simulink model "simrotor1"  (Simulink 10.0)
settings: Solver=ode23tb  StartTime=0.0  StopTime=10.0  RelTol=1e-1  AbsTol=1e-1
undefined symbols (not defined in the file): ar, br, cr, dr, full
libraries: simulink3 x1
settings Model: Creator=bhisma  LastModifiedBy=bhisma  ExtModeTrigMode=oneshot  ExtModeArmWhenConnect=off
settings DataIOCC: SignalLoggingSaveFormat=ModelDataLogs
settings OptimizationCC: BlockReduction=off  BooleanDataType=off  LifeSpan=auto
settings DebuggingCC: SaveWithParameterizedLinksMsg=none  SignalResolutionControl=TryResolveAllWithWarning  MultiTaskDSMMsg=warning  MultiTaskCondExecSysMsg=none  SFUnexpectedBacktrackingDiag=error  SFNoUnconditionalDefaultTransitionDiag=error  SFExecutionAtInitializationDiag=warning  ArithmeticOperatorsInVariantConditions=error
settings HardwareCC: ProdBitPerPointer=64  ProdBitPerSizeT=64  ProdBitPerPtrDiffT=64  ProdLargestAtomicFloat=Float  ProdIntDivRoundTo=Zero  ProdEndianess=LittleEndian  ProdWordSize=64  ProdHWDeviceType=Intel->x86-64 (Windows64)  TargetUnknown=on
settings SFSimCC: SimUseLocalCustomCode=on  CustomCodeUndefinedFunction=FilterOut
settings RTWCC: RTWUseLocalCustomCode=on
settings CodeAppCC: StateflowObjectComments=off
settings GRTTargetCC: TargetLangStandard=C99 (ISO)
settings ConfigComp: CovMetricSettings=dwe  CovHtmlReporting=off  CovSaveCumulativeToWorkspaceVar=off  CovSaveSingleToWorkspaceVar=off

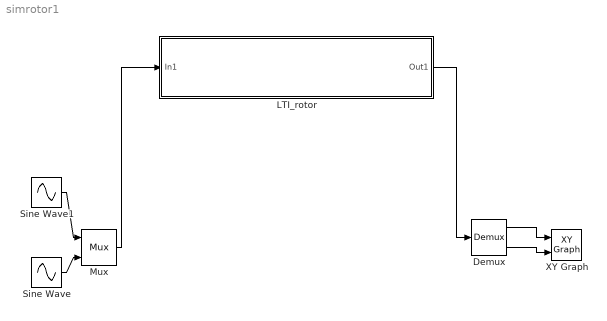
== system simrotor1 ==
  Demux : Demux  Outputs=2
  LTI_rotor : Subsystem  Description=Rotor Linear Model  mask{ModelName=simple2s, W=2500}
      mask prompts: ModelName "Model Template"; W "Speed of Rotation [RPM]"
      mask init:
      | Rot=rotfe(ModelName); [ar,br,cr,dr]=rot2ss(Rot,W*2*pi/60);
      mask Display: disp(ModelName)
  Mux : Mux  Inputs=2
  Sine Wave : Sin  Amplitude=1000  SampleTime=0
  Sine Wave1 : Sin  Amplitude=1000  Phase=pi/2  SampleTime=0
  XY Graph : simulink3/Sinks/XY Graph  xmin=-1  xmax=1  ymin=-1  ymax=1  st=-1
      settings: SourceProductName=Simulink  SourceProductBaseCode=SL
  wires:
  LTI_rotor/1(Out1) -> Demux/1
  Demux/1 -> XY Graph/1
  Demux/2 -> XY Graph/2
  Mux/1 -> LTI_rotor/1(In1)
  Sine Wave/1 -> Mux/2
  Sine Wave1/1 -> Mux/1

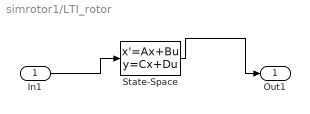
== system simrotor1/LTI_rotor ==
  In1 : Inport
  State-Space : StateSpace  A=full(ar)  B=full(br)  C=full(cr)  D=full(dr)  InitialCondition=0
  Out1 : Outport
  wires:
  In1/1 -> State-Space/1
  State-Space/1 -> Out1/1
